simulink model "SIaD_Tool"  (R2024b)
settings: Solver=ode1  StartTime=0.0  StopTime=Tobs  FixedStep=delta_t  RelTol=1e-3
values from neighbouring files (symbols this model uses):
  delta_t = 25E-6    (= 2.5e-05)    [exe_SIaD.m]
  dist_time = dist_time_f    [FDScanning.m]
  dist_value_0 = Vsignal_dist3    [FDScanning.m]
  dist_value_a = [Isignal_dist3(:,1),zeros(samples_window,1)]    [FDScanning.m]
  dist_value_b = [Isignal_dist3(:,1),zeros(samples_window,1)]    [FDScanning.m]
  dist_value_c = Isignal_dist3    [FDScanning.m]
  dist_value_d = Isignal_dist1    [FDScanning.m]
  dist_value_n = [Vsignal_dist3(:,1),zeros(samples_window,1)]    [FDScanning.m]
  dist_value_p = [Vsignal_dist3(:,1),zeros(samples_window,1)]    [FDScanning.m]
  dist_value_q = [Isignal_dist1(:,1),zeros(samples_window,1)]    [FDScanning.m]
  f0 = fs/Ns    [FDScanning.m]    (also in exe_SIaD.m = 50)
  fd = fd0(n)    [FDScanning.m]
  Id_ss = out.Idq_ss(end-10,1)    [FDScanning.m]    (also in exe_SIaD.m = 0)
  Ipeak = Sbase/Vpeak    [exe_SIaD.m]
  Iq_ss = out.Idq_ss(end-10,2)    [FDScanning.m]    (also in exe_SIaD.m = 0)
  Iss_type = 2    [FDScanning.m]
  phi = (2/3)*pi    (= 2.09439510239)    [FDScanning.m]
  Rsource = 1E-6    (= 1e-06)    [FDScanning.m]
  signal_type = 3    [exe_SIaD.m]
  Vd_ss = out.Vdq_ss(end-10,1)    [FDScanning.m]    (also in exe_SIaD.m = 0)
  Vpeak = (Vbase/sqrt(3))*sqrt(2)    [exe_SIaD.m]
  Vq_ss = out.Vdq_ss(end-10,2)    [FDScanning.m]    (also in exe_SIaD.m = 0)
  Vss_type = 2    [FDScanning.m]
libraries: spsThreePhaseVIMeasurementLib x16, spsControlledCurrentSourceLib x12, spsControlledVoltageSourceLib x12, spsGroundLib x2, spsThreePhaseSeriesRLCBranchLib x2, spsPLL3phLib x1, spspowerguiLib x1
(part 1 of 2)
settings Model: SimulationMode=accelerator  Creator=Luis Angel  LastModifiedBy=GARREYLU
settings OptimizationCC: ReuseModelBlockBuffer=off
settings RTWCC: GPUComputeCapability=3.5

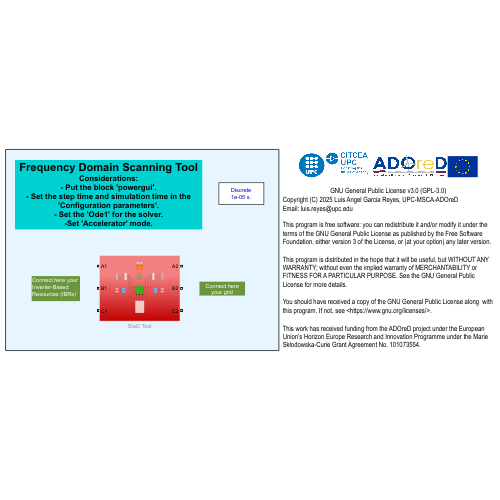
[thumbnail: Simulink's stored preview of the top-level diagram]
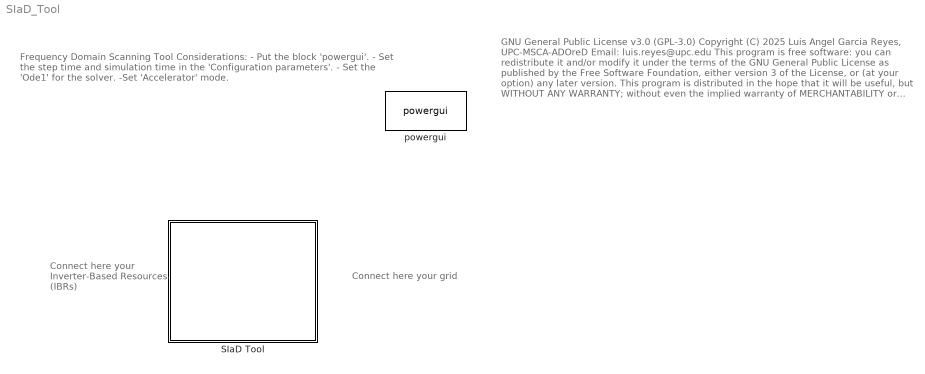
== system SIaD_Tool ==
  note: Frequency Domain Scanning Tool
      | Considerations:
      | - Put the block 'powergui'.
      | - Set the step time and simulation time in the 'Configuration parameters'.
      | - Set the 'Ode1' for the solver.
      | -Set 'Accelerator' mode.
  note: Connect here your Inverter-Based Resources (IBRs)
  note: Connect here your grid
  note: GNU General Public License v3.0 (GPL-3.0)
      | Copyright (C) 2025 Luis Angel Garcia Reyes, UPC-MSCA-ADOreD
      | Email: luis.reyes@upc.edu
      |
      | This program is free software: you can redistribute it and/or modify it under the terms of the GNU General Public License as published by the Free Software Foundation, either version 3 of the License, or (at your option) any later version.
      |
      | This program is distributed in the hope that it will be useful, but WITHOUT ANY WARRANTY; without even the implied warranty of MERCHANTABILITY or FITNESS FOR A PARTICULAR PURPOSE. See the GNU General Public License for more details.
      |
      | You should have received a copy of the GNU General Public License along with this program. If not, see <https://www.gnu.org/licenses/>.
      |
      | This work has received funding from the ADOreD project under the European Union’s Horizon Europe Research and Innovation Programme under the Marie Skłodowska-Curie Grant Agreement No. 101073554.
  SIaD Tool : Subsystem
  powergui : spspowerguiLib/powergui  Priority=1  SimulationMode=Discrete  SampleTime=delta_t  frequency=60  Iterations=50  frequencyindice=0  Pbase=100e6  ErrMax=1e-4  UnitsV=kV  UnitsW=MW  buscounter=0  FunctionMessages=off  echomessages=off  EnableUseOfTLC=off  CurrentSourceSwitches=off  DisableSnubberDevices=off  DisableRonSwitches=off  DisableVfSwitches=off  DisplayEquations=off  AutomaticDiscreteSolvers=off  SolverType=Tustin/Backward Euler (TBE)  Interpol=off  ExternalGateDelay=off  methode=off  Ts=100  x0status=blocks  SPID=on  SwTol=0  HookPort=off  NonlinearTolerance=1e-4  nMaxIteration=100  ContinueOnMaxIteration=off  RestoreLinks=warning  ResistiveCurrentMeasurement=off  Frange=[0:2:500]  Ylog=off  Xlog=on  ShowGrid=off  save=off  variable=ZData  structure=0  ZoomFFT=off  StartTime=0.0  cycles=1  DisplayStyle=1  fundamental=60  FreqAxis=off  MaxFrequency=1000  frequencyindicesteady=1  RmsSteady=1  display=off

== system SIaD_Tool/SIaD Tool ==
  Decoupled State : Subsystem
      settings: PortSchema="{\"entries\":[{\"content\":{\"sides\":[{\"content\":{\"connectorIds\":[\"LConn1\",\"LConn2\",\"LConn3\"]},\"type\":\"ConnectorPlacement.EquallySpacedRectSide\",\"uuid\":\"d0026cad-bf69-43aa-99db-8cc8562f1524\"},{\"content\":{\"side\":\"RIGHT\"},\"type\":\"ConnectorPlacement.EquallySpacedRectSide\",\"uuid\":\"64b8bea8-dfd1-490d-8772-f15621dca227\"},{\"content\":{\"connectorIds\":[\"LConn4\",\"LConn5\",\"LConn6\"],\"side\":\"TOP\"},\"type\":\"ConnectorPlacement.EquallySpacedRectSide\",\"uuid\":\"5c20e442-7542-4d44-8051-809eca545f48\"},{\"content\":{\"connectorIds\":[\"RConn1\",\"RConn2\",\"RConn3\"],\"side\":\"BOTTOM\"},\"type\":\"ConnectorPlacement.EquallySpacedRectSide\",\"uuid\":\"0dac49be-ef95-43f1-976a-782473b2e343\"}]},\"type\":\"ConnectorPlacement.EquallySpacedConnector\",\"uuid\":\"aff4678d-8b0f-4c58-9998-b2e98e043de0\"}],\"packageUris\":[\"http://schema.mathworks.com/mf0/Connector/R2020b\"],\"version\":\"1.0\"}"
  Frequency Scanner : Subsystem
  Normal State : Subsystem  Commented=on
  Steady State : Subsystem  Commented=on
  System 1 : Subsystem
  System 1 Meas : spsThreePhaseVIMeasurementLib/Three-Phase V-I Measurement  VoltageMeasurement=phase-to-ground  SetLabelV=on  LabelV=Vabc1  Vpu=off  VpuLL=off  CurrentMeasurement=yes  SetLabelI=on  LabelI=Iabc1  Ipu=off  Pbase=100e6  Vbase=500e3  OutputType=Complex  PhasorSimulation=off  PSBequivalent=0
  System 2 : Subsystem
  System 2 Meas : spsThreePhaseVIMeasurementLib/Three-Phase V-I Measurement  VoltageMeasurement=phase-to-ground  SetLabelV=on  LabelV=Vabc2  Vpu=off  VpuLL=off  CurrentMeasurement=yes  SetLabelI=on  LabelI=Iabc2  Ipu=off  Pbase=100e6  Vbase=500e3  OutputType=Complex  PhasorSimulation=off  PSBequivalent=0
  A2 : PMIOPort  Side=Left
  B2 : PMIOPort  Port=2  Side=Left
  C2 : PMIOPort  Port=3  Side=Left
  A1 : PMIOPort  Port=4  Side=Right
  B1 : PMIOPort  Port=5  Side=Right
  C1 : PMIOPort  Port=6  Side=Right
  wires:
  [Vabc1] -> Steady State/1(Voltage)
  [Iabc1] -> Steady State/2(Current)
  [Iabc1] -> System 1/2(Current1)
  [Vabc1] -> System 1/1(Voltage1)
  [Vabc2] -> System 2/1(Voltage2)
  [Iabc2] -> System 2/2(Current2)
  connections:
  Normal State/LConn1 -- System 1 Meas/LConn1 -- Decoupled State/LConn6
  Normal State/RConn3 -- System 2 Meas/LConn3 -- Decoupled State/RConn1
  Decoupled State/LConn5 -- System 1 Meas/LConn2 -- Normal State/LConn2
  Normal State/LConn3 -- System 1 Meas/LConn3 -- Decoupled State/LConn4
  Normal State/RConn1 -- System 2 Meas/LConn1 -- Decoupled State/RConn3
  Normal State/RConn2 -- System 2 Meas/LConn2 -- Decoupled State/RConn2
  Decoupled State/LConn1 -- Frequency Scanner/LConn1
  Decoupled State/LConn2 -- Frequency Scanner/LConn2
  Decoupled State/LConn3 -- Frequency Scanner/LConn3
  System 1 Meas/RConn1 -- A1/RConn1
  System 1 Meas/RConn2 -- B1/RConn1
  System 1 Meas/RConn3 -- C1/RConn1
  System 2 Meas/RConn1 -- A2/RConn1
  System 2 Meas/RConn2 -- B2/RConn1
  System 2 Meas/RConn3 -- C2/RConn1

== system SIaD_Tool/SIaD Tool/Decoupled State ==
  Three-Phase V-I Measurement7 : spsThreePhaseVIMeasurementLib/Three-Phase V-I Measurement  VoltageMeasurement=no  SetLabelV=on  LabelV=Vabc  Vpu=off  VpuLL=off  CurrentMeasurement=no  SetLabelI=on  LabelI=Iabc  Ipu=off  Pbase=100e6  Vbase=500e3  OutputType=Complex  PhasorSimulation=off  PSBequivalent=0
  Three-Phase V-I Measurement8 : spsThreePhaseVIMeasurementLib/Three-Phase V-I Measurement  VoltageMeasurement=no  SetLabelV=on  LabelV=Vabc  Vpu=off  VpuLL=off  CurrentMeasurement=no  SetLabelI=on  LabelI=Iabc  Ipu=off  Pbase=100e6  Vbase=500e3  OutputType=Complex  PhasorSimulation=off  PSBequivalent=0
  A : PMIOPort  Side=Left
  B : PMIOPort  Port=2  Side=Left
  C : PMIOPort  Port=3  Side=Left
  S1c : PMIOPort  Port=4  Side=Left
  S1b : PMIOPort  Port=5  Side=Left
  S1a : PMIOPort  Port=6  Side=Left
  S2c : PMIOPort  Port=7  Side=Right
  S2b : PMIOPort  Port=8  Side=Right
  S2a : PMIOPort  Port=9  Side=Right
  connections:
  S1a/RConn1 -- S2a/RConn1 -- Three-Phase V-I Measurement7/LConn1
  A/RConn1 -- Three-Phase V-I Measurement8/RConn1
  B/RConn1 -- Three-Phase V-I Measurement8/RConn2
  C/RConn1 -- Three-Phase V-I Measurement8/RConn3
  Three-Phase V-I Measurement8/LConn1 -- Three-Phase V-I Measurement7/RConn1
  Three-Phase V-I Measurement8/LConn2 -- Three-Phase V-I Measurement7/RConn2
  Three-Phase V-I Measurement8/LConn3 -- Three-Phase V-I Measurement7/RConn3
  S1b/RConn1 -- S2b/RConn1 -- Three-Phase V-I Measurement7/LConn2
  S1c/RConn1 -- S2c/RConn1 -- Three-Phase V-I Measurement7/LConn3

== system SIaD_Tool/SIaD Tool/Frequency Scanner ==
  note: Current perturbation method
  note: Voltage perturbation method
  Current Strategy : Subsystem  Commented=on
  Three-Phase V-I Measurement1 : spsThreePhaseVIMeasurementLib/Three-Phase V-I Measurement  VoltageMeasurement=no  SetLabelV=on  LabelV=Vabc  Vpu=off  VpuLL=off  CurrentMeasurement=no  SetLabelI=on  LabelI=Iabc  Ipu=off  Pbase=100e6  Vbase=500e3  OutputType=Complex  PhasorSimulation=off  PSBequivalent=0
  Three-Phase V-I Measurement3 : spsThreePhaseVIMeasurementLib/Three-Phase V-I Measurement  VoltageMeasurement=no  SetLabelV=on  LabelV=Vabc  Vpu=off  VpuLL=off  CurrentMeasurement=no  SetLabelI=on  LabelI=Iabc  Ipu=off  Pbase=100e6  Vbase=500e3  OutputType=Complex  PhasorSimulation=off  PSBequivalent=0
  Voltage Strategy : Subsystem
  a : PMIOPort  Side=Left
  b : PMIOPort  Port=2  Side=Left
  c : PMIOPort  Port=3  Side=Left
  connections:
  Three-Phase V-I Measurement3/LConn2 -- Current Strategy/LConn2
  Three-Phase V-I Measurement3/RConn3 -- Three-Phase V-I Measurement1/RConn3 -- c/RConn1
  Three-Phase V-I Measurement3/RConn1 -- a/RConn1 -- Three-Phase V-I Measurement1/RConn1
  Three-Phase V-I Measurement3/LConn1 -- Current Strategy/LConn1
  Three-Phase V-I Measurement3/RConn2 -- Three-Phase V-I Measurement1/RConn2 -- b/RConn1
  Three-Phase V-I Measurement3/LConn3 -- Current Strategy/LConn3
  Three-Phase V-I Measurement1/LConn1 -- Voltage Strategy/RConn1
  Three-Phase V-I Measurement1/LConn3 -- Voltage Strategy/RConn3
  Three-Phase V-I Measurement1/LConn2 -- Voltage Strategy/RConn2

== system SIaD_Tool/SIaD Tool/Normal State ==
  Three-Phase V-I Measurement7 : spsThreePhaseVIMeasurementLib/Three-Phase V-I Measurement  VoltageMeasurement=no  SetLabelV=on  LabelV=Vabc  Vpu=off  VpuLL=off  CurrentMeasurement=no  SetLabelI=on  LabelI=Iabc  Ipu=off  Pbase=100e6  Vbase=500e3  OutputType=Complex  PhasorSimulation=off  PSBequivalent=0
  Three-Phase V-I Measurement8 : spsThreePhaseVIMeasurementLib/Three-Phase V-I Measurement  VoltageMeasurement=no  SetLabelV=on  LabelV=Vabc  Vpu=off  VpuLL=off  CurrentMeasurement=no  SetLabelI=on  LabelI=Iabc  Ipu=off  Pbase=100e6  Vbase=500e3  OutputType=Complex  PhasorSimulation=off  PSBequivalent=0
  a : PMIOPort  Side=Right
  A : PMIOPort  Port=2  Side=Left
  b : PMIOPort  Port=3  Side=Right
  B : PMIOPort  Port=4  Side=Left
  c : PMIOPort  Port=5  Side=Right
  C : PMIOPort  Port=6  Side=Left
  connections:
  Three-Phase V-I Measurement7/LConn2 -- Three-Phase V-I Measurement8/RConn2
  Three-Phase V-I Measurement7/RConn2 -- b/RConn1
  Three-Phase V-I Measurement7/LConn3 -- Three-Phase V-I Measurement8/RConn3
  Three-Phase V-I Measurement7/LConn1 -- Three-Phase V-I Measurement8/RConn1
  Three-Phase V-I Measurement7/RConn3 -- c/RConn1
  Three-Phase V-I Measurement8/LConn1 -- A/RConn1
  Three-Phase V-I Measurement8/LConn3 -- C/RConn1
  Three-Phase V-I Measurement7/RConn1 -- a/RConn1
  Three-Phase V-I Measurement8/LConn2 -- B/RConn1

== system SIaD_Tool/SIaD Tool/Steady State ==
  note: Voltage measurements
  note: Voltage measurements
  Voltage : Inport
  Current : Inport  Port=2
  Demux1 : Demux  Outputs=3
  Demux2 : Demux  Outputs=3
  Fortescue Transformation : Subsystem
  Fortescue Transformation1 : Subsystem
  Mux1 : Mux  Inputs=2
  Mux2 : Mux  Inputs=2
  PLL (3ph) : spsPLL3phLib/PLL (3ph)  Fmin=45  Par_Init=[0, f0]  ParK=[180, 3200, 1]  TcD=1e-4  MaxRateChangeFreq=12  FilterCutOffFreq=25  Ts=delta_t  AGC=on
  Park Transform1 : Subsystem
  Park Transform2 : Subsystem
  Terminator1 : Terminator
  Terminator2 : Terminator
  Terminator4 : Terminator
  To Workspace1 : ToWorkspace  VariableName=Vabc_ss  SampleTime=-1
  To Workspace2 : ToWorkspace  VariableName=Iabc_ss  SampleTime=-1
  To Workspace22 : ToWorkspace  VariableName=Vdq_ss  SampleTime=-1
  To Workspace3 : ToWorkspace  VariableName=Idq_ss  SampleTime=-1
  To Workspace4 : ToWorkspace  VariableName=I0pn_ss  SampleTime=-1
  To Workspace7 : ToWorkspace  VariableName=V0pn_ss  SampleTime=-1
  wires:
  Demux2/3 -> Terminator2/1
  PLL (3ph)/2 -> [wt_ss], Park Transform2/2(wt)
  Voltage/1 -> Fortescue Transformation/1(ABC), PLL (3ph)/1, Park Transform2/1(ABC), To Workspace1/1
  PLL (3ph)/1 -> Terminator1/1
  Mux2/1 -> To Workspace22/1
  Fortescue Transformation/1(0PN) -> To Workspace7/1
  Demux2/1 -> Mux2/1
  Park Transform2/1(qd0) -> Demux2/1
  Demux2/2 -> Mux2/2
  Park Transform1/1(qd0) -> Demux1/1
  Demux1/1 -> Mux1/1
  Fortescue Transformation1/1(0PN) -> To Workspace4/1
  Mux1/1 -> To Workspace3/1
  Demux1/3 -> Terminator4/1
  Current/1 -> Fortescue Transformation1/1(ABC), To Workspace2/1, Park Transform1/1(ABC)
  Demux1/2 -> Mux1/2
  [wt_ss] -> Park Transform1/2(wt)

== system SIaD_Tool/SIaD Tool/System 1 ==
  Voltage1 : Inport
  Current1 : Inport  Port=2
  0pn Sequence : Subsystem  Commented=on
  ABC Sequence : Subsystem
  dq0 Sequence : Subsystem  Commented=on
  wires:
  Voltage1/1 -> 0pn Sequence/1(Vabc), dq0 Sequence/1(Vabc), ABC Sequence/1(Vabc)
  Current1/1 -> 0pn Sequence/2(Iabc), dq0 Sequence/2(Iabc), ABC Sequence/2(Iabc)

== system SIaD_Tool/SIaD Tool/System 2 ==
  Voltage2 : Inport
  Current2 : Inport  Port=2
  0pn Sequence : Subsystem  Commented=on
  ABC Sequence : Subsystem
  dq0 Sequence : Subsystem  Commented=on
  wires:
  Voltage2/1 -> 0pn Sequence/1(Vabc), dq0 Sequence/1(Vabc), ABC Sequence/1(Vabc)
  Current2/1 -> 0pn Sequence/2(Iabc), dq0 Sequence/2(Iabc), ABC Sequence/2(Iabc)

== system SIaD_Tool/SIaD Tool/Frequency Scanner/Current Strategy ==
  note: qd0 scan
  note: Fundamental source
  note: pn0 scan
  note: ABC scan
  ABCdisturbance2 : Subsystem
  Current Fundamental Source : Subsystem
      settings: PortSchema="{\"entries\":[{\"content\":{\"sides\":[{\"content\":{\"connectorIds\":[\"Out1\"]},\"type\":\"ConnectorPlacement.EquallySpacedRectSide\",\"uuid\":\"2a4baa29-0316-4256-b4e1-e3ef1d370b3b\"},{\"content\":{\"connectorIds\":[\"RConn1\",\"RConn2\",\"RConn3\"],\"side\":\"RIGHT\"},\"type\":\"ConnectorPlacement.EquallySpacedRectSide\",\"uuid\":\"3108b85a-ac52-49ed-83a6-d77923640585\"},{\"content\":{\"connectorIds\":[],\"side\":\"TOP\"},\"type\":\"ConnectorPlacement.EquallySpacedRectSide\",\"uuid\":\"4093502e-3b8b-4232-aa57-5a461ca3ca63\"},{\"content\":{\"connectorIds\":[\"RConn4\"],\"side\":\"BOTTOM\"},\"type\":\"ConnectorPlacement.EquallySpacedRectSide\",\"uuid\":\"50c06102-7582-4746-a571-3f791f943454\"}]},\"type\":\"ConnectorPlacement.EquallySpacedConnector\",\"uuid\":\"209f4db4-fe77-48a5-84ae-6773984a343b\"}],\"packageUris\":[\"http://schema.mathworks.com/mf0/Connector/R2020b\"],\"version\":\"1.0\"}"
  Three-Phase V-I Measurement2 : spsThreePhaseVIMeasurementLib/Three-Phase V-I Measurement  VoltageMeasurement=no  SetLabelV=on  LabelV=Vabc  Vpu=off  VpuLL=off  CurrentMeasurement=no  SetLabelI=on  LabelI=Iabc  Ipu=off  Pbase=100e6  Vbase=500e3  OutputType=Complex  PhasorSimulation=off  PSBequivalent=0
  pn0disturbance2 : Subsystem  Commented=on
  qd0disturbance2 : Subsystem  Commented=on
      settings: PortSchema="{\"entries\":[{\"content\":{\"sides\":[{\"content\":{\"connectorIds\":[\"LConn1\",\"LConn2\",\"LConn3\",\"LConn4\"]},\"type\":\"ConnectorPlacement.EquallySpacedRectSide\",\"uuid\":\"96b61a08-e73c-4bf9-b44c-8e6d57b8ef4a\"},{\"content\":{\"connectorIds\":[\"RConn1\",\"RConn2\",\"RConn3\"],\"side\":\"RIGHT\"},\"type\":\"ConnectorPlacement.EquallySpacedRectSide\",\"uuid\":\"3a0e4222-9b60-4a58-9d08-3b159ebff1b9\"},{\"content\":{\"connectorIds\":[\"In1\"],\"side\":\"TOP\"},\"type\":\"ConnectorPlacement.EquallySpacedRectSide\",\"uuid\":\"61af63da-f353-4270-b8c9-89c35459604e\"}]},\"type\":\"ConnectorPlacement.EquallySpacedConnector\",\"uuid\":\"24d596f4-e3d4-42a2-b524-8b1140a91bdb\"}],\"packageUris\":[\"http://schema.mathworks.com/mf0/Connector/R2020b\"],\"version\":\"1.0\"}"
  Aout : PMIOPort  Side=Left
  Bout : PMIOPort  Port=2  Side=Left
  Cout : PMIOPort  Port=3  Side=Left
  tag scope: theta_ref=global
  wires:
  [theta_ref] -> qd0disturbance2/1(theta)
  Current Fundamental Source/1(theta) -> [theta_ref]
  connections:
  pn0disturbance2/RConn1 -- Aout/RConn1 -- ABCdisturbance2/RConn1 -- qd0disturbance2/RConn1
  pn0disturbance2/RConn2 -- Bout/RConn1 -- ABCdisturbance2/RConn2 -- qd0disturbance2/RConn2
  Current Fundamental Source/RConn2 -- Three-Phase V-I Measurement2/LConn2
  Three-Phase V-I Measurement2/RConn2 -- pn0disturbance2/LConn2 -- ABCdisturbance2/LConn2 -- qd0disturbance2/LConn2
  Current Fundamental Source/RConn3 -- Three-Phase V-I Measurement2/LConn3
  pn0disturbance2/RConn3 -- Cout/RConn1 -- ABCdisturbance2/RConn3 -- qd0disturbance2/RConn3
  Three-Phase V-I Measurement2/RConn1 -- pn0disturbance2/LConn1 -- ABCdisturbance2/LConn1 -- qd0disturbance2/LConn1
  Current Fundamental Source/RConn4 -- pn0disturbance2/LConn4 -- ABCdisturbance2/LConn4 -- qd0disturbance2/LConn4
  Three-Phase V-I Measurement2/RConn3 -- pn0disturbance2/LConn3 -- ABCdisturbance2/LConn3 -- qd0disturbance2/LConn3
  Current Fundamental Source/RConn1 -- Three-Phase V-I Measurement2/LConn1

== system SIaD_Tool/SIaD Tool/Frequency Scanner/Voltage Strategy ==
  note: Fundamental source
  note: pn0 scan
  note: ABC scan
  note: qd0 scan
  ABCdisturbance : Subsystem
  Three-Phase V-I Measurement : spsThreePhaseVIMeasurementLib/Three-Phase V-I Measurement  VoltageMeasurement=no  SetLabelV=on  LabelV=Vabc  Vpu=off  VpuLL=off  CurrentMeasurement=no  SetLabelI=on  LabelI=Iabc  Ipu=off  Pbase=100e6  Vbase=500e3  OutputType=Complex  PhasorSimulation=off  PSBequivalent=0
  Voltage Fundamental Source : Subsystem
      settings: PortSchema="{\"entries\":[{\"content\":{\"sides\":[{\"content\":{\"connectorIds\":[\"Out1\"]},\"type\":\"ConnectorPlacement.EquallySpacedRectSide\",\"uuid\":\"3dbf8d23-22ab-4ddc-ae4a-19197e180312\"},{\"content\":{\"connectorIds\":[\"RConn1\",\"RConn2\",\"RConn3\"],\"side\":\"RIGHT\"},\"type\":\"ConnectorPlacement.EquallySpacedRectSide\",\"uuid\":\"df914263-db35-4888-aa99-5dec7a54c6e0\"},{\"content\":{\"connectorIds\":[],\"side\":\"TOP\"},\"type\":\"ConnectorPlacement.EquallySpacedRectSide\",\"uuid\":\"815bd59d-9d4f-4637-8c0a-95368e7d07f9\"}]},\"type\":\"ConnectorPlacement.EquallySpacedConnector\",\"uuid\":\"b7ffca83-a6f6-4340-8cfa-6aec16cec0d1\"}],\"packageUris\":[\"http://schema.mathworks.com/mf0/Connector/R2020b\"],\"version\":\"1.0\"}"
  pn0disturbance : Subsystem  Commented=on
  qd0disturbance : Subsystem  Commented=on
      settings: PortSchema="{\"entries\":[{\"content\":{\"sides\":[{\"content\":{\"connectorIds\":[\"LConn1\",\"LConn2\",\"LConn3\"]},\"type\":\"ConnectorPlacement.EquallySpacedRectSide\",\"uuid\":\"96b61a08-e73c-4bf9-b44c-8e6d57b8ef4a\"},{\"content\":{\"connectorIds\":[\"RConn1\",\"RConn2\",\"RConn3\"],\"side\":\"RIGHT\"},\"type\":\"ConnectorPlacement.EquallySpacedRectSide\",\"uuid\":\"3a0e4222-9b60-4a58-9d08-3b159ebff1b9\"},{\"content\":{\"connectorIds\":[\"In1\"],\"side\":\"TOP\"},\"type\":\"ConnectorPlacement.EquallySpacedRectSide\",\"uuid\":\"61af63da-f353-4270-b8c9-89c35459604e\"}]},\"type\":\"ConnectorPlacement.EquallySpacedConnector\",\"uuid\":\"24d596f4-e3d4-42a2-b524-8b1140a91bdb\"}],\"packageUris\":[\"http://schema.mathworks.com/mf0/Connector/R2020b\"],\"version\":\"1.0\"}"
  Aout : PMIOPort  Side=Right
  Bout : PMIOPort  Port=2  Side=Right
  Cout : PMIOPort  Port=3  Side=Right
  tag scope: theta_ref=global
  wires:
  Voltage Fundamental Source/1(theta) -> [theta_ref]
  [theta_ref] -> qd0disturbance/1(theta)
  connections:
  ABCdisturbance/RConn2 -- Bout/RConn1 -- pn0disturbance/RConn2 -- qd0disturbance/RConn2
  Voltage Fundamental Source/RConn1 -- Three-Phase V-I Measurement/LConn1
  qd0disturbance/LConn3 -- ABCdisturbance/LConn3 -- Three-Phase V-I Measurement/RConn3 -- pn0disturbance/LConn3
  ABCdisturbance/RConn1 -- Aout/RConn1 -- pn0disturbance/RConn1 -- qd0disturbance/RConn1
  Voltage Fundamental Source/RConn2 -- Three-Phase V-I Measurement/LConn2
  Voltage Fundamental Source/RConn3 -- Three-Phase V-I Measurement/LConn3
  ABCdisturbance/RConn3 -- Cout/RConn1 -- pn0disturbance/RConn3 -- qd0disturbance/RConn3
  qd0disturbance/LConn1 -- ABCdisturbance/LConn1 -- Three-Phase V-I Measurement/RConn1 -- pn0disturbance/LConn1
  qd0disturbance/LConn2 -- ABCdisturbance/LConn2 -- Three-Phase V-I Measurement/RConn2 -- pn0disturbance/LConn2

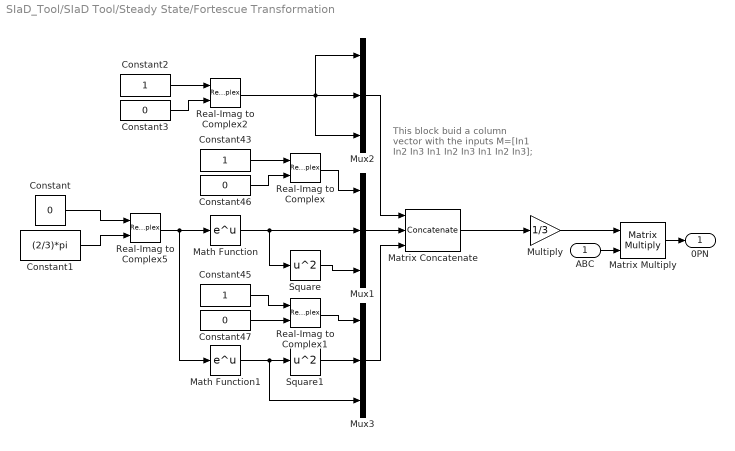
== system SIaD_Tool/SIaD Tool/Steady State/Fortescue Transformation ==
  note: This block buid a column vector with the inputs
      | M=[In1 In2 In3
      |       In1 In2 In3
      |       In1 In2 In3];
  ABC : Inport
  Constant{,3,46..47} (4 alike) : Constant  Value=0
  Constant1 : Constant  Value=(2/3)*pi
  Constant2 : Constant
  Constant43 : Constant
  Constant45 : Constant
  Math Function : Math
  Math Function1 : Math
  Matrix Concatenate : Concatenate  NumInputs=3  Mode=Multidimensional array  ConcatenateDimension=2
  Matrix Multiply : Product  Multiplication=Matrix(*)
  Multiply : Gain  Gain=1/3
  Mux1 : Mux  Inputs=3
  Mux2 : Mux  Inputs=3
  Mux3 : Mux  Inputs=3
  Real-Imag to Complex{,1..2,5} (4 alike) : RealImagToComplex
  Square : Math  Operator=square
  Square1 : Math  Operator=square
  0PN : Outport
  wires:
  Square/1 -> Mux1/3
  Math Function/1 -> Mux1/2, Square/1
  Real-Imag to Complex1/1 -> Mux3/1
  Square1/1 -> Mux3/2
  Multiply/1 -> Matrix Multiply/1
  Math Function1/1 -> Square1/1, Mux3/3
  Mux3/1 -> Matrix Concatenate/3
  Constant45/1 -> Real-Imag to Complex1/1
  Matrix Concatenate/1 -> Multiply/1
  Real-Imag to Complex2/1 -> Mux2/2, Mux2/1, Mux2/3
  Real-Imag to Complex5/1 -> Math Function1/1, Math Function/1
  ABC/1 -> Matrix Multiply/2
  Mux2/1 -> Matrix Concatenate/1
  Constant47/1 -> Real-Imag to Complex1/2
  Mux1/1 -> Matrix Concatenate/2
  Real-Imag to Complex/1 -> Mux1/1
  Constant46/1 -> Real-Imag to Complex/2
  Constant43/1 -> Real-Imag to Complex/1
  Matrix Multiply/1 -> 0PN/1
  Constant1/1 -> Real-Imag to Complex5/2
  Constant/1 -> Real-Imag to Complex5/1
  Constant2/1 -> Real-Imag to Complex2/1
  Constant3/1 -> Real-Imag to Complex2/2

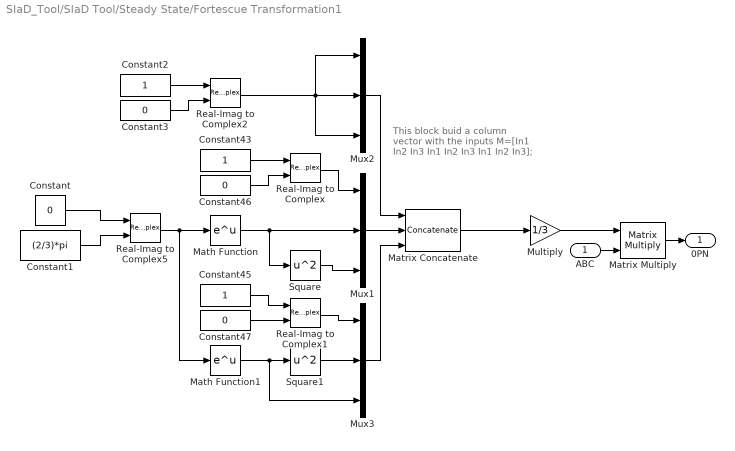
== system SIaD_Tool/SIaD Tool/Steady State/Fortescue Transformation1 ==
  note: This block buid a column vector with the inputs
      | M=[In1 In2 In3
      |       In1 In2 In3
      |       In1 In2 In3];
  ABC : Inport
  Constant{,3,46..47} (4 alike) : Constant  Value=0
  Constant1 : Constant  Value=(2/3)*pi
  Constant2 : Constant
  Constant43 : Constant
  Constant45 : Constant
  Math Function : Math
  Math Function1 : Math
  Matrix Concatenate : Concatenate  NumInputs=3  Mode=Multidimensional array  ConcatenateDimension=2
  Matrix Multiply : Product  Multiplication=Matrix(*)
  Multiply : Gain  Gain=1/3
  Mux1 : Mux  Inputs=3
  Mux2 : Mux  Inputs=3
  Mux3 : Mux  Inputs=3
  Real-Imag to Complex{,1..2,5} (4 alike) : RealImagToComplex
  Square : Math  Operator=square
  Square1 : Math  Operator=square
  0PN : Outport
  wires:
  Square/1 -> Mux1/3
  Math Function/1 -> Mux1/2, Square/1
  Real-Imag to Complex1/1 -> Mux3/1
  Square1/1 -> Mux3/2
  Multiply/1 -> Matrix Multiply/1
  Math Function1/1 -> Square1/1, Mux3/3
  Mux3/1 -> Matrix Concatenate/3
  Constant45/1 -> Real-Imag to Complex1/1
  Matrix Concatenate/1 -> Multiply/1
  Real-Imag to Complex2/1 -> Mux2/2, Mux2/1, Mux2/3
  Real-Imag to Complex5/1 -> Math Function1/1, Math Function/1
  ABC/1 -> Matrix Multiply/2
  Mux2/1 -> Matrix Concatenate/1
  Constant47/1 -> Real-Imag to Complex1/2
  Mux1/1 -> Matrix Concatenate/2
  Real-Imag to Complex/1 -> Mux1/1
  Constant46/1 -> Real-Imag to Complex/2
  Constant43/1 -> Real-Imag to Complex/1
  Matrix Multiply/1 -> 0PN/1
  Constant1/1 -> Real-Imag to Complex5/2
  Constant/1 -> Real-Imag to Complex5/1
  Constant2/1 -> Real-Imag to Complex2/1
  Constant3/1 -> Real-Imag to Complex2/2

== system SIaD_Tool/SIaD Tool/Steady State/Park Transform1 ==
  ABC : Inport
  wt : Inport  Port=2
  Constant : Constant  Value=1/2
  Constant1 : Constant  Value=1/2
  Constant2 : Constant  Value=1/2
  Constant3 : Constant  Value=(2*pi)/3
  Constant4 : Constant  Value=(2*pi)/3
  Cos : Trigonometry  Operator=cos
  Cos1 : Trigonometry  Operator=cos
  Cos2 : Trigonometry  Operator=cos
  Gain : Gain  Gain=2/3
  Matrix Concatenate : Concatenate  NumInputs=3  Mode=Multidimensional array  ConcatenateDimension=2
  Matrix Multiply : Product  Multiplication=Matrix(*)
  Mux : Mux  Inputs=3
  Mux1 : Mux  Inputs=3
  Mux2 : Mux  Inputs=3
  Sin : Trigonometry
  Sin1 : Trigonometry
  Sin2 : Trigonometry
  Sum : Sum  Inputs=|+-
  Sum1 : Sum  Inputs=|++
  qd0 : Outport
  wires:
  Sum/1 -> Sin1/1, Cos1/1
  Constant1/1 -> Mux1/3
  Sin2/1 -> Mux2/2
  Gain/1 -> Matrix Multiply/1
  Cos/1 -> Mux/1
  Constant3/1 -> Sum/2
  wt/1 -> Cos/1, Sin/1, Sum/1, Sum1/1
  Sum1/1 -> Sin2/1, Cos2/1
  Mux1/1 -> Matrix Concatenate/2
  Sin/1 -> Mux/2
  Constant4/1 -> Sum1/2
  Constant2/1 -> Mux2/3
  Mux2/1 -> Matrix Concatenate/3
  Cos2/1 -> Mux2/1
  Constant/1 -> Mux/3
  Matrix Concatenate/1 -> Gain/1
  Cos1/1 -> Mux1/1
  Sin1/1 -> Mux1/2
  Mux/1 -> Matrix Concatenate/1
  ABC/1 -> Matrix Multiply/2
  Matrix Multiply/1 -> qd0/1

== system SIaD_Tool/SIaD Tool/Steady State/Park Transform2 ==
  ABC : Inport
  wt : Inport  Port=2
  Constant : Constant  Value=1/2
  Constant1 : Constant  Value=1/2
  Constant2 : Constant  Value=1/2
  Constant3 : Constant  Value=(2*pi)/3
  Constant4 : Constant  Value=(2*pi)/3
  Cos : Trigonometry  Operator=cos
  Cos1 : Trigonometry  Operator=cos
  Cos2 : Trigonometry  Operator=cos
  Gain : Gain  Gain=2/3
  Matrix Concatenate : Concatenate  NumInputs=3  Mode=Multidimensional array  ConcatenateDimension=2
  Matrix Multiply : Product  Multiplication=Matrix(*)
  Mux : Mux  Inputs=3
  Mux1 : Mux  Inputs=3
  Mux2 : Mux  Inputs=3
  Sin : Trigonometry
  Sin1 : Trigonometry
  Sin2 : Trigonometry
  Sum : Sum  Inputs=|+-
  Sum1 : Sum  Inputs=|++
  qd0 : Outport
  wires:
  Sum/1 -> Sin1/1, Cos1/1
  Constant1/1 -> Mux1/3
  Sin2/1 -> Mux2/2
  Gain/1 -> Matrix Multiply/1
  Cos/1 -> Mux/1
  Constant3/1 -> Sum/2
  wt/1 -> Cos/1, Sin/1, Sum/1, Sum1/1
  Sum1/1 -> Sin2/1, Cos2/1
  Mux1/1 -> Matrix Concatenate/2
  Sin/1 -> Mux/2
  Constant4/1 -> Sum1/2
  Constant2/1 -> Mux2/3
  Mux2/1 -> Matrix Concatenate/3
  Cos2/1 -> Mux2/1
  Constant/1 -> Mux/3
  Matrix Concatenate/1 -> Gain/1
  Cos1/1 -> Mux1/1
  Sin1/1 -> Mux1/2
  Mux/1 -> Matrix Concatenate/1
  ABC/1 -> Matrix Multiply/2
  Matrix Multiply/1 -> qd0/1

== system SIaD_Tool/SIaD Tool/System 1/0pn Sequence ==
  Vabc : Inport
  Iabc : Inport  Port=2
  Fortescue Transformation : Subsystem
  Fortescue Transformation1 : Subsystem
  To Workspace53 : ToWorkspace  VariableName=I0pn1  SampleTime=-1
  To Workspace7 : ToWorkspace  VariableName=V0pn1  SampleTime=-1
  wires:
  Fortescue Transformation1/1(0PN) -> To Workspace53/1
  Iabc/1 -> Fortescue Transformation1/1(ABC)
  Fortescue Transformation/1(0PN) -> To Workspace7/1
  Vabc/1 -> Fortescue Transformation/1(ABC)

== system SIaD_Tool/SIaD Tool/System 1/ABC Sequence ==
  note: ABC sequence
  Vabc : Inport
  Iabc : Inport  Port=2
  To Workspace4 : ToWorkspace  VariableName=Vabc1  SampleTime=-1
  To Workspace5 : ToWorkspace  VariableName=Iabc1  SampleTime=-1
  wires:
  Vabc/1 -> To Workspace4/1
  Iabc/1 -> To Workspace5/1

== system SIaD_Tool/SIaD Tool/System 1/dq0 Sequence ==
  Vabc : Inport
  Iabc : Inport  Port=2
  Demux2 : Demux  Outputs=3
  Demux3 : Demux  Outputs=3
  Mux1 : Mux  Inputs=2
  Mux2 : Mux  Inputs=2
  Park Transform : Subsystem
  Park Transform1 : Subsystem
  Scope : Scope
  Scope1 : Scope
  Terminator1 : Terminator
  Terminator2 : Terminator
  To Workspace22 : ToWorkspace  VariableName=Vqd1  SampleTime=-1
  To Workspace23 : ToWorkspace  VariableName=Iqd1  SampleTime=-1
  wires:
  Mux1/1 -> Scope1/1, To Workspace23/1
  Demux3/2 -> Mux1/2
  Demux2/3 -> Terminator2/1
  Park Transform/1(qd0) -> Demux2/1
  [theta_ref] -> Park Transform1/2(wt)
  Demux3/1 -> Mux1/1
  Demux3/3 -> Terminator1/1
  [theta_ref] -> Park Transform/2(wt)
  Demux2/1 -> Mux2/1
  Mux2/1 -> Scope/1, To Workspace22/1
  Demux2/2 -> Mux2/2
  Park Transform1/1(qd0) -> Demux3/1
  Iabc/1 -> Park Transform1/1(ABC)
  Vabc/1 -> Park Transform/1(ABC)

== system SIaD_Tool/SIaD Tool/System 2/0pn Sequence ==
  Vabc : Inport
  Iabc : Inport  Port=2
  Fortescue Transformation : Subsystem
  Fortescue Transformation1 : Subsystem
  To Workspace53 : ToWorkspace  VariableName=I0pn2  SampleTime=-1
  To Workspace7 : ToWorkspace  VariableName=V0pn2  SampleTime=-1
  wires:
  Fortescue Transformation1/1(0PN) -> To Workspace53/1
  Iabc/1 -> Fortescue Transformation1/1(ABC)
  Fortescue Transformation/1(0PN) -> To Workspace7/1
  Vabc/1 -> Fortescue Transformation/1(ABC)

== system SIaD_Tool/SIaD Tool/System 2/ABC Sequence ==
  note: ABC sequence
  Vabc : Inport
  Iabc : Inport  Port=2
  To Workspace4 : ToWorkspace  VariableName=Vabc2  SampleTime=-1
  To Workspace5 : ToWorkspace  VariableName=Iabc2  SampleTime=-1
  wires:
  Vabc/1 -> To Workspace4/1
  Iabc/1 -> To Workspace5/1

== system SIaD_Tool/SIaD Tool/System 2/dq0 Sequence ==
  Vabc : Inport
  Iabc : Inport  Port=2
  Demux2 : Demux  Outputs=3
  Demux3 : Demux  Outputs=3
  Mux1 : Mux  Inputs=2
  Mux2 : Mux  Inputs=2
  Park Transform : Subsystem
  Park Transform1 : Subsystem
  Terminator1 : Terminator
  Terminator2 : Terminator
  To Workspace22 : ToWorkspace  VariableName=Vqd2  SampleTime=-1
  To Workspace23 : ToWorkspace  VariableName=Iqd2  SampleTime=-1
  wires:
  Mux1/1 -> To Workspace23/1
  Demux3/2 -> Mux1/2
  Demux2/3 -> Terminator2/1
  Park Transform/1(qd0) -> Demux2/1
  [theta_ref] -> Park Transform1/2(wt)
  Demux3/1 -> Mux1/1
  Demux3/3 -> Terminator1/1
  [theta_ref] -> Park Transform/2(wt)
  Demux2/1 -> Mux2/1
  Mux2/1 -> To Workspace22/1
  Demux2/2 -> Mux2/2
  Park Transform1/1(qd0) -> Demux3/1
  Iabc/1 -> Park Transform1/1(ABC)
  Vabc/1 -> Park Transform/1(ABC)

== system SIaD_Tool/SIaD Tool/Frequency Scanner/Current Strategy/ABCdisturbance2 ==
  Constant : Constant  Value=signal_type
  Controlled Current Source : spsControlledCurrentSourceLib/Controlled Current Source  Initialize=off  Source_Type=AC  Amplitude=0  Phase=0  Frequency=0  Measurements=None
  Controlled Current Source1 : spsControlledCurrentSourceLib/Controlled Current Source  Initialize=off  Source_Type=AC  Amplitude=0  Phase=0  Frequency=0  Measurements=None
  Controlled Current Source2 : spsControlledCurrentSourceLib/Controlled Current Source  Initialize=off  Source_Type=AC  Amplitude=0  Phase=0  Frequency=0  Measurements=None
  Demux : Demux  Outputs=3
  From8 : From
  Goto4 : Goto
  Multi-tone : Subsystem  Commented=on
  Single-tone : Subsystem
  Switch : Switch  Criteria=u2 > Threshold  Threshold=1  SaturateOnIntegerOverflow=off  InputSameDT=off
  Three-Phase V-I Measurement3 : spsThreePhaseVIMeasurementLib/Three-Phase V-I Measurement  VoltageMeasurement=no  SetLabelV=on  LabelV=Vabc4  Vpu=off  VpuLL=off  CurrentMeasurement=no  SetLabelI=on  LabelI=Iabc4  Ipu=off  Pbase=100e6  Vbase=500e3  OutputType=Complex  PhasorSimulation=off  PSBequivalent=0
  Ain : PMIOPort  Side=Left
  Bin : PMIOPort  Port=2  Side=Left
  Cin : PMIOPort  Port=3  Side=Left
  Aout : PMIOPort  Port=4  Side=Right
  Bout : PMIOPort  Port=5  Side=Right
  Cout : PMIOPort  Port=6  Side=Right
  GND : PMIOPort  Port=7  Side=Left
  wires:
  [C] -> Controlled Current Source2/1
  [B] -> Controlled Current Source1/1
  From8/1 -> Controlled Current Source/1
  Constant/1 -> Switch/2
  Multi-tone/1(ABC) -> Switch/1
  Demux/1 -> Goto4/1
  Demux/2 -> [B]
  Demux/3 -> [C]
  Switch/1 -> Demux/1
  Single-tone/1(ABC) -> Switch/3
  connections:
  Controlled Current Source1/LConn1 -- GND/RConn1 -- Controlled Current Source2/LConn1 -- Controlled Current Source/LConn1
  Controlled Current Source/RConn1 -- Three-Phase V-I Measurement3/LConn1 -- Ain/RConn1
  Controlled Current Source2/RConn1 -- Three-Phase V-I Measurement3/LConn3 -- Cin/RConn1
  Controlled Current Source1/RConn1 -- Three-Phase V-I Measurement3/LConn2 -- Bin/RConn1
  Three-Phase V-I Measurement3/RConn1 -- Aout/RConn1
  Three-Phase V-I Measurement3/RConn2 -- Bout/RConn1
  Three-Phase V-I Measurement3/RConn3 -- Cout/RConn1

== system SIaD_Tool/SIaD Tool/Frequency Scanner/Current Strategy/Current Fundamental Source ==
  Controlled Current Source : spsControlledCurrentSourceLib/Controlled Current Source  Initialize=off  Source_Type=AC  Amplitude=0  Phase=0  Frequency=0  Measurements=None
  Controlled Current Source1 : spsControlledCurrentSourceLib/Controlled Current Source  Initialize=off  Source_Type=AC  Amplitude=0  Phase=0  Frequency=0  Measurements=None
  Controlled Current Source2 : spsControlledCurrentSourceLib/Controlled Current Source  Initialize=off  Source_Type=AC  Amplitude=0  Phase=0  Frequency=0  Measurements=None
  Grid Currents1 : Subsystem
  Ground : spsGroundLib/Ground  LConnTagsString=a
  Three-Phase Series RLC Branch : spsThreePhaseSeriesRLCBranchLib/Three-Phase Series RLC Branch  LConnTagsString=A|B|C  RConnTagsString=A|B|C  BranchType=R  Resistance=1/Rsource  Inductance=1e-3  Capacitance=1e-6  Measurements=None
  VzA : PMIOPort  Side=Right
  VzB : PMIOPort  Port=2  Side=Right
  VzC : PMIOPort  Port=3  Side=Right
  GND : PMIOPort  Port=4  Side=Right
  theta : Outport
  wires:
  Grid Currents1/3(IC) -> Controlled Current Source/1
  Grid Currents1/2(IB) -> Controlled Current Source1/1
  Grid Currents1/1(IA) -> Controlled Current Source2/1
  Grid Currents1/4(theta) -> theta/1
  connections:
  Controlled Current Source2/RConn1 -- Three-Phase Series RLC Branch/LConn1 -- VzA/RConn1
  Controlled Current Source1/RConn1 -- Three-Phase Series RLC Branch/LConn2 -- VzB/RConn1
  Controlled Current Source/RConn1 -- Three-Phase Series RLC Branch/LConn3 -- VzC/RConn1
  Ground/LConn1 -- Controlled Current Source/LConn1 -- Controlled Current Source1/LConn1 -- Controlled Current Source2/LConn1 -- Three-Phase Series RLC Branch/RConn3 -- Three-Phase Series RLC Branch/RConn2 -- Three-Phase Series RLC Branch/RConn1 -- GND/RConn1

== system SIaD_Tool/SIaD Tool/Frequency Scanner/Current Strategy/pn0disturbance2 ==
  Constant : Constant  Value=signal_type
  Controlled Current Source : spsControlledCurrentSourceLib/Controlled Current Source  Initialize=off  Source_Type=AC  Amplitude=0  Phase=0  Frequency=0  Measurements=None
  Controlled Current Source1 : spsControlledCurrentSourceLib/Controlled Current Source  Initialize=off  Source_Type=AC  Amplitude=0  Phase=0  Frequency=0  Measurements=None
  Controlled Current Source2 : spsControlledCurrentSourceLib/Controlled Current Source  Initialize=off  Source_Type=AC  Amplitude=0  Phase=0  Frequency=0  Measurements=None
  Demux : Demux  Outputs=3
  From1 : From
  Goto1 : Goto
  Multi-tone : Subsystem
  Single-tone : Subsystem  Commented=on
  Switch : Switch  Criteria=u2 > Threshold  Threshold=1  SaturateOnIntegerOverflow=off  InputSameDT=off
  Three-Phase V-I Measurement3 : spsThreePhaseVIMeasurementLib/Three-Phase V-I Measurement  VoltageMeasurement=no  SetLabelV=on  LabelV=Vabc6  Vpu=off  VpuLL=off  CurrentMeasurement=no  SetLabelI=on  LabelI=Iabc6  Ipu=off  Pbase=100e6  Vbase=500e3  OutputType=Complex  PhasorSimulation=off  PSBequivalent=0
  Ain : PMIOPort  Side=Left
  Bin : PMIOPort  Port=2  Side=Left
  Cin : PMIOPort  Port=3  Side=Left
  Aout : PMIOPort  Port=4  Side=Right
  Bout : PMIOPort  Port=5  Side=Right
  Cout : PMIOPort  Port=6  Side=Right
  GND : PMIOPort  Port=7  Side=Left
  wires:
  [B] -> Controlled Current Source1/1
  [C] -> Controlled Current Source2/1
  From1/1 -> Controlled Current Source/1
  Multi-tone/1(ABC) -> Switch/1
  Demux/1 -> Goto1/1
  Demux/3 -> [C]
  Constant/1 -> Switch/2
  Single-tone/1(ABC) -> Switch/3
  Switch/1 -> Demux/1
  Demux/2 -> [B]
  connections:
  Cin/RConn1 -- Three-Phase V-I Measurement3/LConn3 -- Controlled Current Source2/RConn1
  Controlled Current Source1/LConn1 -- GND/RConn1 -- Controlled Current Source2/LConn1 -- Controlled Current Source/LConn1
  Ain/RConn1 -- Three-Phase V-I Measurement3/LConn1 -- Controlled Current Source/RConn1
  Bin/RConn1 -- Three-Phase V-I Measurement3/LConn2 -- Controlled Current Source1/RConn1
  Three-Phase V-I Measurement3/RConn3 -- Cout/RConn1
  Three-Phase V-I Measurement3/RConn2 -- Bout/RConn1
  Three-Phase V-I Measurement3/RConn1 -- Aout/RConn1

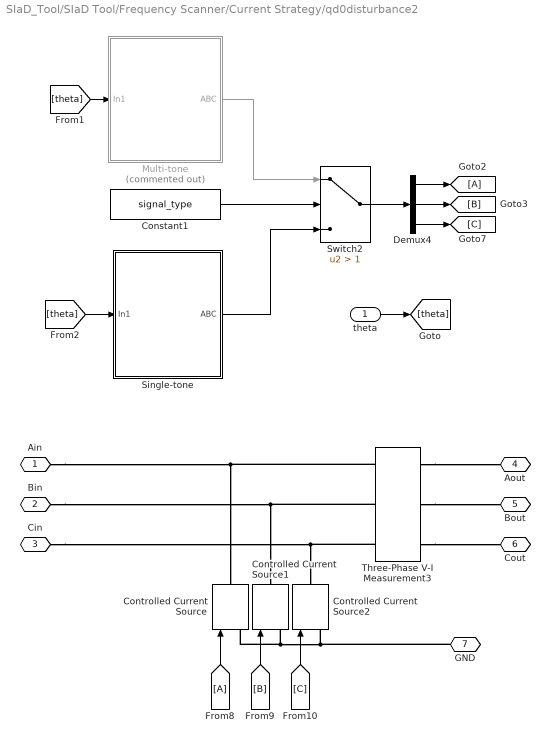
== system SIaD_Tool/SIaD Tool/Frequency Scanner/Current Strategy/qd0disturbance2 ==
  theta : Inport
  Constant1 : Constant  Value=signal_type
  Controlled Current Source : spsControlledCurrentSourceLib/Controlled Current Source  Initialize=off  Source_Type=AC  Amplitude=0  Phase=0  Frequency=0  Measurements=None
  Controlled Current Source1 : spsControlledCurrentSourceLib/Controlled Current Source  Initialize=off  Source_Type=AC  Amplitude=0  Phase=0  Frequency=0  Measurements=None
  Controlled Current Source2 : spsControlledCurrentSourceLib/Controlled Current Source  Initialize=off  Source_Type=AC  Amplitude=0  Phase=0  Frequency=0  Measurements=None
  Demux4 : Demux  Outputs=3
  From8 : From
  Goto2 : Goto
  Multi-tone : Subsystem  Commented=on
  Single-tone : Subsystem
  Switch2 : Switch  Criteria=u2 > Threshold  Threshold=1  SaturateOnIntegerOverflow=off  InputSameDT=off
  Three-Phase V-I Measurement3 : spsThreePhaseVIMeasurementLib/Three-Phase V-I Measurement  VoltageMeasurement=no  SetLabelV=on  LabelV=Vabc5  Vpu=off  VpuLL=off  CurrentMeasurement=no  SetLabelI=on  LabelI=Iabc5  Ipu=off  Pbase=100e6  Vbase=500e3  OutputType=Complex  PhasorSimulation=off  PSBequivalent=0
  Ain : PMIOPort  Side=Left
  Bin : PMIOPort  Port=2  Side=Left
  Cin : PMIOPort  Port=3  Side=Left
  Aout : PMIOPort  Port=4  Side=Right
  Bout : PMIOPort  Port=5  Side=Right
  Cout : PMIOPort  Port=6  Side=Right
  GND : PMIOPort  Port=7  Side=Left
  wires:
  theta/1 -> [theta]
  From8/1 -> Controlled Current Source/1
  [C] -> Controlled Current Source2/1
  [B] -> Controlled Current Source1/1
  Constant1/1 -> Switch2/2
  Multi-tone/1(ABC) -> Switch2/1
  [theta] -> Single-tone/1(In1)
  Switch2/1 -> Demux4/1
  Single-tone/1(ABC) -> Switch2/3
  Demux4/1 -> Goto2/1
  Demux4/2 -> [B]
  [theta] -> Multi-tone/1(In1)
  Demux4/3 -> [C]
  connections:
  Controlled Current Source1/LConn1 -- GND/RConn1 -- Controlled Current Source2/LConn1 -- Controlled Current Source/LConn1
  Ain/RConn1 -- Three-Phase V-I Measurement3/LConn1 -- Controlled Current Source/RConn1
  Bin/RConn1 -- Three-Phase V-I Measurement3/LConn2 -- Controlled Current Source1/RConn1
  Cin/RConn1 -- Three-Phase V-I Measurement3/LConn3 -- Controlled Current Source2/RConn1
  Three-Phase V-I Measurement3/RConn1 -- Aout/RConn1
  Three-Phase V-I Measurement3/RConn2 -- Bout/RConn1
  Three-Phase V-I Measurement3/RConn3 -- Cout/RConn1

== system SIaD_Tool/SIaD Tool/Frequency Scanner/Voltage Strategy/ABCdisturbance ==
  Constant : Constant  Value=signal_type
  Controlled Voltage Source1 : spsControlledVoltageSourceLib/Controlled Voltage Source  Initialize=off  Source_Type=DC  Amplitude=0  Phase=0  Frequency=0  Measurements=None
  Controlled Voltage Source2 : spsControlledVoltageSourceLib/Controlled Voltage Source  Initialize=off  Source_Type=DC  Amplitude=0  Phase=0  Frequency=0  Measurements=None
  Controlled Voltage Source6 : spsControlledVoltageSourceLib/Controlled Voltage Source  Initialize=off  Source_Type=DC  Amplitude=0  Phase=0  Frequency=0  Measurements=None
  Demux : Demux  Outputs=3
  From2 : From
  Goto4 : Goto
  Multi-tone : Subsystem  Commented=on
  Single-tone : Subsystem
  Switch : Switch  Criteria=u2 > Threshold  Threshold=1  SaturateOnIntegerOverflow=off  InputSameDT=off
  Three-Phase V-I Measurement : spsThreePhaseVIMeasurementLib/Three-Phase V-I Measurement  VoltageMeasurement=no  SetLabelV=on  LabelV=Vabc  Vpu=off  VpuLL=off  CurrentMeasurement=no  SetLabelI=off  LabelI=Iabc  Ipu=off  Pbase=100e6  Vbase=500e3  OutputType=Complex  PhasorSimulation=off  PSBequivalent=0
  Ain1 : PMIOPort  Side=Left
  Bin1 : PMIOPort  Port=2  Side=Left
  Cin1 : PMIOPort  Port=3  Side=Left
  Aout : PMIOPort  Port=4  Side=Right
  Bout : PMIOPort  Port=5  Side=Right
  Cout : PMIOPort  Port=6  Side=Right
  wires:
  [C] -> Controlled Voltage Source6/1
  From2/1 -> Controlled Voltage Source1/1
  [B] -> Controlled Voltage Source2/1
  Multi-tone/1(ABC) -> Switch/1
  Demux/3 -> [C]
  Constant/1 -> Switch/2
  Demux/1 -> Goto4/1
  Demux/2 -> [B]
  Single-tone/1(ABC) -> Switch/3
  Switch/1 -> Demux/1
  connections:
  Bin1/RConn1 -- Controlled Voltage Source2/LConn1
  Controlled Voltage Source1/LConn1 -- Ain1/RConn1
  Cin1/RConn1 -- Controlled Voltage Source6/LConn1
  Three-Phase V-I Measurement/LConn1 -- Controlled Voltage Source1/RConn1
  Three-Phase V-I Measurement/LConn2 -- Controlled Voltage Source2/RConn1
  Three-Phase V-I Measurement/LConn3 -- Controlled Voltage Source6/RConn1
  Three-Phase V-I Measurement/RConn3 -- Cout/RConn1
  Three-Phase V-I Measurement/RConn2 -- Bout/RConn1
  Three-Phase V-I Measurement/RConn1 -- Aout/RConn1

== system SIaD_Tool/SIaD Tool/Frequency Scanner/Voltage Strategy/Voltage Fundamental Source ==
  Controlled Voltage Source1 : spsControlledVoltageSourceLib/Controlled Voltage Source  Initialize=off  Source_Type=DC  Amplitude=0  Phase=0  Frequency=0  Measurements=None
  Controlled Voltage Source2 : spsControlledVoltageSourceLib/Controlled Voltage Source  Initialize=off  Source_Type=DC  Amplitude=0  Phase=0  Frequency=0  Measurements=None
  Controlled Voltage Source3 : spsControlledVoltageSourceLib/Controlled Voltage Source  Initialize=off  Source_Type=DC  Amplitude=0  Phase=0  Frequency=0  Measurements=None
  Grid Voltages : Subsystem
  Ground : spsGroundLib/Ground  LConnTagsString=a
  Three-Phase Series RLC Branch : spsThreePhaseSeriesRLCBranchLib/Three-Phase Series RLC Branch  LConnTagsString=A|B|C  RConnTagsString=A|B|C  BranchType=R  Resistance=Rsource  Inductance=1e-3  Capacitance=1e-6  Measurements=None
  VzA : PMIOPort  Side=Right
  VzB : PMIOPort  Port=2  Side=Right
  VzC : PMIOPort  Port=3  Side=Right
  theta : Outport
  wires:
  Grid Voltages/3(VC) -> Controlled Voltage Source3/1
  Grid Voltages/2(VB) -> Controlled Voltage Source2/1
  Grid Voltages/1(VA) -> Controlled Voltage Source1/1
  Grid Voltages/4(theta) -> theta/1
  connections:
  Controlled Voltage Source2/LConn1 -- Controlled Voltage Source1/LConn1 -- Controlled Voltage Source3/LConn1 -- Ground/LConn1
  Three-Phase Series RLC Branch/RConn1 -- Controlled Voltage Source1/RConn1
  Three-Phase Series RLC Branch/RConn2 -- Controlled Voltage Source2/RConn1
  Three-Phase Series RLC Branch/RConn3 -- Controlled Voltage Source3/RConn1
  Three-Phase Series RLC Branch/LConn3 -- VzC/RConn1
  Three-Phase Series RLC Branch/LConn2 -- VzB/RConn1
  Three-Phase Series RLC Branch/LConn1 -- VzA/RConn1

== system SIaD_Tool/SIaD Tool/Frequency Scanner/Voltage Strategy/pn0disturbance ==
  Constant : Constant  Value=signal_type
  Controlled Voltage Source1 : spsControlledVoltageSourceLib/Controlled Voltage Source  Initialize=off  Source_Type=DC  Amplitude=0  Phase=0  Frequency=0  Measurements=None
  Controlled Voltage Source2 : spsControlledVoltageSourceLib/Controlled Voltage Source  Initialize=off  Source_Type=DC  Amplitude=0  Phase=0  Frequency=0  Measurements=None
  Controlled Voltage Source6 : spsControlledVoltageSourceLib/Controlled Voltage Source  Initialize=off  Source_Type=DC  Amplitude=0  Phase=0  Frequency=0  Measurements=None
  Demux : Demux  Outputs=3
  From3 : From
  Goto1 : Goto
  Multi-tone : Subsystem
  Single-tone : Subsystem  Commented=on
  Switch : Switch  Criteria=u2 > Threshold  Threshold=1  SaturateOnIntegerOverflow=off  InputSameDT=off
  Three-Phase V-I Measurement3 : spsThreePhaseVIMeasurementLib/Three-Phase V-I Measurement  VoltageMeasurement=no  SetLabelV=on  LabelV=Vabc3  Vpu=off  VpuLL=off  CurrentMeasurement=no  SetLabelI=on  LabelI=Iabc3  Ipu=off  Pbase=100e6  Vbase=500e3  OutputType=Complex  PhasorSimulation=off  PSBequivalent=0
  Ain : PMIOPort  Side=Left
  Bin : PMIOPort  Port=2  Side=Left
  Cin : PMIOPort  Port=3  Side=Left
  Aout : PMIOPort  Port=4  Side=Right
  Bout : PMIOPort  Port=5  Side=Right
  Cout : PMIOPort  Port=6  Side=Right
  wires:
  [B] -> Controlled Voltage Source2/1
  From3/1 -> Controlled Voltage Source1/1
  [C] -> Controlled Voltage Source6/1
  Switch/1 -> Demux/1
  Single-tone/1(ABC) -> Switch/3
  Demux/3 -> [C]
  Multi-tone/1(ABC) -> Switch/1
  Demux/1 -> Goto1/1
  Demux/2 -> [B]
  Constant/1 -> Switch/2
  connections:
  Controlled Voltage Source1/LConn1 -- Ain/RConn1
  Cin/RConn1 -- Controlled Voltage Source6/LConn1
  Bin/RConn1 -- Controlled Voltage Source2/LConn1
  Three-Phase V-I Measurement3/LConn1 -- Controlled Voltage Source1/RConn1
  Three-Phase V-I Measurement3/LConn2 -- Controlled Voltage Source2/RConn1
  Three-Phase V-I Measurement3/LConn3 -- Controlled Voltage Source6/RConn1
  Three-Phase V-I Measurement3/RConn1 -- Aout/RConn1
  Three-Phase V-I Measurement3/RConn2 -- Bout/RConn1
  Three-Phase V-I Measurement3/RConn3 -- Cout/RConn1

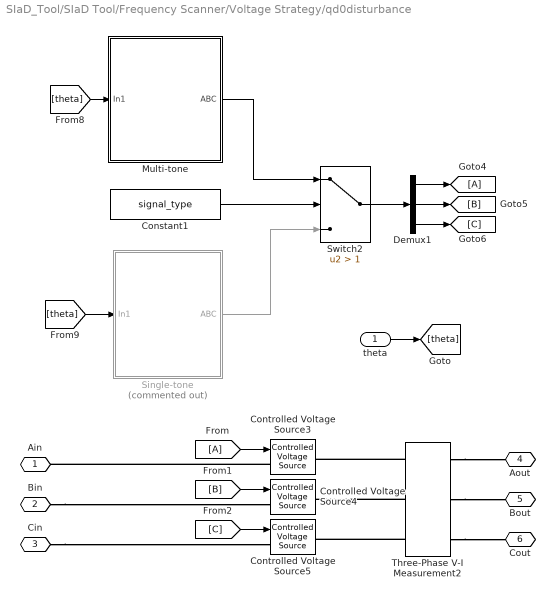
== system SIaD_Tool/SIaD Tool/Frequency Scanner/Voltage Strategy/qd0disturbance ==
  theta : Inport
  Constant1 : Constant  Value=signal_type
  Controlled Voltage Source3 : spsControlledVoltageSourceLib/Controlled Voltage Source  Initialize=off  Source_Type=DC  Amplitude=0  Phase=0  Frequency=0  Measurements=None
  Controlled Voltage Source4 : spsControlledVoltageSourceLib/Controlled Voltage Source  Initialize=off  Source_Type=DC  Amplitude=0  Phase=0  Frequency=0  Measurements=None
  Controlled Voltage Source5 : spsControlledVoltageSourceLib/Controlled Voltage Source  Initialize=off  Source_Type=DC  Amplitude=0  Phase=0  Frequency=0  Measurements=None
  Demux1 : Demux  Outputs=3
  From : From
  Goto4 : Goto
  Multi-tone : Subsystem
  Single-tone : Subsystem  Commented=on
  Switch2 : Switch  Criteria=u2 > Threshold  Threshold=1  SaturateOnIntegerOverflow=off  InputSameDT=off
  Three-Phase V-I Measurement2 : spsThreePhaseVIMeasurementLib/Three-Phase V-I Measurement  VoltageMeasurement=no  SetLabelV=on  LabelV=Vabc2  Vpu=off  VpuLL=off  CurrentMeasurement=no  SetLabelI=on  LabelI=Iabc2  Ipu=off  Pbase=100e6  Vbase=500e3  OutputType=Complex  PhasorSimulation=off  PSBequivalent=0
  Ain : PMIOPort  Side=Left
  Bin : PMIOPort  Port=2  Side=Left
  Cin : PMIOPort  Port=3  Side=Left
  Aout : PMIOPort  Port=4  Side=Right
  Bout : PMIOPort  Port=5  Side=Right
  Cout : PMIOPort  Port=6  Side=Right
  wires:
  From/1 -> Controlled Voltage Source3/1
  [B] -> Controlled Voltage Source4/1
  [C] -> Controlled Voltage Source5/1
  theta/1 -> [theta]
  Switch2/1 -> Demux1/1
  Single-tone/1(ABC) -> Switch2/3
  Multi-tone/1(ABC) -> Switch2/1
  Constant1/1 -> Switch2/2
  [theta] -> Single-tone/1(In1)
  Demux1/3 -> [C]
  Demux1/1 -> Goto4/1
  Demux1/2 -> [B]
  [theta] -> Multi-tone/1(In1)
  connections:
  Controlled Voltage Source3/LConn1 -- Ain/RConn1
  Bin/RConn1 -- Controlled Voltage Source4/LConn1
  Cin/RConn1 -- Controlled Voltage Source5/LConn1
  Three-Phase V-I Measurement2/LConn1 -- Controlled Voltage Source3/RConn1
  Three-Phase V-I Measurement2/LConn2 -- Controlled Voltage Source4/RConn1
  Three-Phase V-I Measurement2/LConn3 -- Controlled Voltage Source5/RConn1
  Three-Phase V-I Measurement2/RConn1 -- Aout/RConn1
  Three-Phase V-I Measurement2/RConn2 -- Bout/RConn1
  Three-Phase V-I Measurement2/RConn3 -- Cout/RConn1

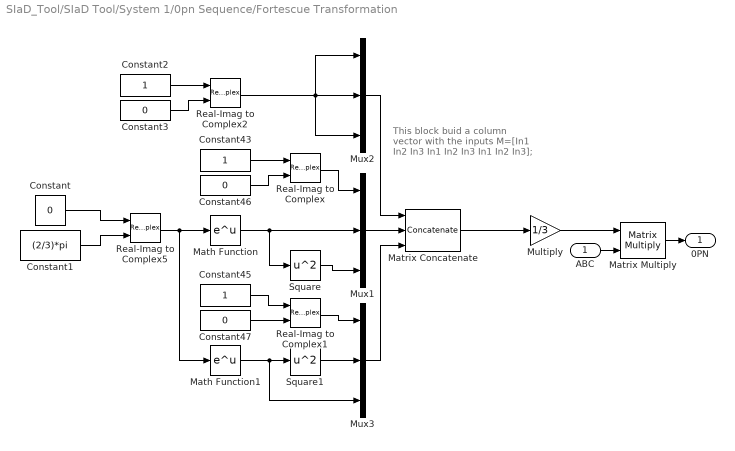
== system SIaD_Tool/SIaD Tool/System 1/0pn Sequence/Fortescue Transformation ==
  note: This block buid a column vector with the inputs
      | M=[In1 In2 In3
      |       In1 In2 In3
      |       In1 In2 In3];
  ABC : Inport
  Constant{,3,46..47} (4 alike) : Constant  Value=0
  Constant1 : Constant  Value=(2/3)*pi
  Constant2 : Constant
  Constant43 : Constant
  Constant45 : Constant
  Math Function : Math
  Math Function1 : Math
  Matrix Concatenate : Concatenate  NumInputs=3  Mode=Multidimensional array  ConcatenateDimension=2
  Matrix Multiply : Product  Multiplication=Matrix(*)
  Multiply : Gain  Gain=1/3
  Mux1 : Mux  Inputs=3
  Mux2 : Mux  Inputs=3
  Mux3 : Mux  Inputs=3
  Real-Imag to Complex{,1..2,5} (4 alike) : RealImagToComplex
  Square : Math  Operator=square
  Square1 : Math  Operator=square
  0PN : Outport
  wires:
  Square/1 -> Mux1/3
  Math Function/1 -> Mux1/2, Square/1
  Real-Imag to Complex1/1 -> Mux3/1
  Square1/1 -> Mux3/2
  Multiply/1 -> Matrix Multiply/1
  Math Function1/1 -> Square1/1, Mux3/3
  Mux3/1 -> Matrix Concatenate/3
  Constant45/1 -> Real-Imag to Complex1/1
  Matrix Concatenate/1 -> Multiply/1
  Real-Imag to Complex2/1 -> Mux2/2, Mux2/1, Mux2/3
  Real-Imag to Complex5/1 -> Math Function1/1, Math Function/1
  ABC/1 -> Matrix Multiply/2
  Mux2/1 -> Matrix Concatenate/1
  Constant47/1 -> Real-Imag to Complex1/2
  Mux1/1 -> Matrix Concatenate/2
  Real-Imag to Complex/1 -> Mux1/1
  Constant46/1 -> Real-Imag to Complex/2
  Constant43/1 -> Real-Imag to Complex/1
  Matrix Multiply/1 -> 0PN/1
  Constant1/1 -> Real-Imag to Complex5/2
  Constant/1 -> Real-Imag to Complex5/1
  Constant2/1 -> Real-Imag to Complex2/1
  Constant3/1 -> Real-Imag to Complex2/2
